simulink model "fm_reciver_01"  (R2021b)
settings: Solver=VariableStepAuto  StartTime=0.0  StopTime=0.5  RelTol=1e-3
libraries: dspsnks4 x1, commsdrhw_v2 x1
settings Model: Creator=Rajeev Ranjan  LastModifiedBy=Rajeev Ranjan

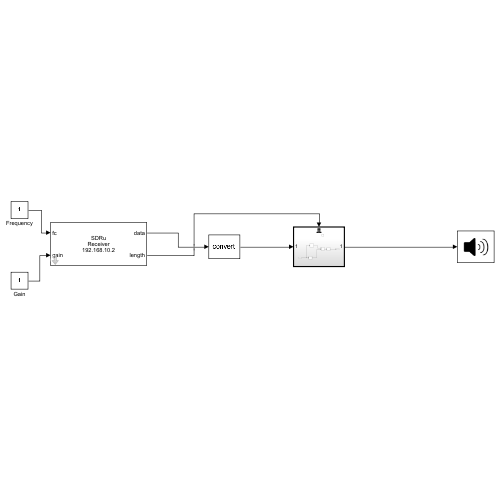
[thumbnail: Simulink's stored preview of the top-level diagram]
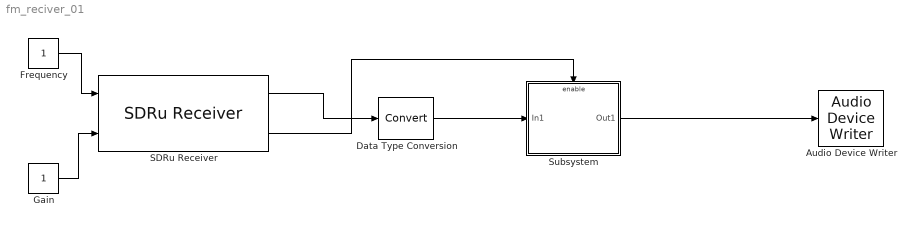
== system fm_reciver_01 ==
  Audio Device Writer : dspsnks4/Audio Device Writer  Driver=DirectSound  Device=Default  InheritSampleRate=on  SampleRate=44100  BitDepth=16-bit integer  BufferSize=4096  NumBuffers=10  DefaultOutputChannelMapping=on  OutputChannelMapping=1:2  OutputNumUnderrunSamples=off  DriverIdx=1  DeviceWarnFlag=''
  Data Type Conversion : DataTypeConversion
  Frequency : Constant
  Gain : Constant
  SDRu Receiver : commsdrhw_v2/SDRu Receiver  rxtx=rx  initializeIPAddress=0  devMap=10  USRP2_IP=192.168.10.2  USRP_IP_X300=192.168.10.2  USRP_IP_X310=No devices found  USRP_IP_N300=192.168.10.2  USRP_IP_N310=192.168.10.2  USRP_IP_N320=192.168.10.2  USRP_serialNumB200=No devices found  USRP_serialNumB210=3136D21  platform=N200/N210/USRP2  prevPlatform=N200/N210/USRP2  lastIPAddressPopup=192.168.10.2  USRP_ID=192.168.10.2  LastIPAddress=192.168.10.2  IsTwinRXDaughterboard=off  EnableTwinRXPhaseSync=off  losrc=0  ChannelMapping=1  centerFrequencySrc=Input port  centerFrequency=2.45e9  loOffsetSrc=Dialog  loOffset=0  gainSrc=Input port  gain=32  PPSSource=Internal  EnableGPSLock=off  EnsureSyncGPSTime=off  clockSource=Internal  EnableRefLock=off  masterClkRateParam=100e6  masterClkRateB200=32e6  masterClkRateB210=32e6  masterClkRateX300=200e6  masterClkRateX310=200e6  masterClkRateN300=125e6  masterClkRateN310=125e6  masterClkRateN320=200e6  masterClkRate=100e6  masterClkRateTwinRX=200e6  decimInterpSrc=Dialog  decimInterpPort=512  lastDecimSource=Dialog  decimInterp=500  USRP2_IP_NUM=[49 57 50 46 49 54 56 46 49 48 46 50]  sampleRate=200000  sampleTime=500/100000000  TransportDataType=int16  overrunUnderrunPort=off  outputDatatype=single  frameLength=4000  HOST_DATA_PORT=0  HOST_CONTROL_PORT=0  USRP2_DATA_PORT=0  USRP2_CONTROL_PORT=0  bufferMode=Continuous streaming  EnableBurstMode=on  NumFramesInBurst=100
      settings: SourceProductBaseCode=USRP
  Subsystem : Subsystem
  wires:
  Data Type Conversion/1 -> Subsystem/1(In1)
  Subsystem/1(Out1) -> Audio Device Writer/1
  SDRu Receiver/1 -> Data Type Conversion/1
  SDRu Receiver/2 -> Subsystem/Enable
  Frequency/1 -> SDRu Receiver/1
  Gain/1 -> SDRu Receiver/2

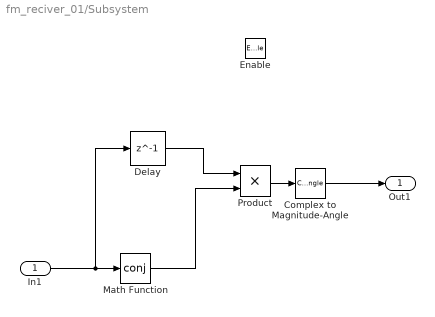
== system fm_reciver_01/Subsystem ==
  In1 : Inport
  Enable : EnablePort
  Complex to Magnitude-Angle : ComplexToMagnitudeAngle  Output=Angle
  Delay : Delay  DelayLength=1  InitialCondition=0  InputProcessing=Columns as channels (frame based)
  Math Function : Math  Operator=conj  SaturateOnIntegerOverflow=on
  Product : Product
  Out1 : Outport
  wires:
  Complex to Magnitude-Angle/1 -> Out1/1
  Math Function/1 -> Product/2
  In1/1 -> Delay/1, Math Function/1
  Product/1 -> Complex to Magnitude-Angle/1
  Delay/1 -> Product/1
